simulink library "atomicSubSystem"  (R2023a)
settings: Solver=VariableStepAuto  StartTime=0.0  StopTime=10.0  RelTol=1e-3
libraries: $bdroot x1
settings Model: Creator=Franz  LastModifiedBy=Franz

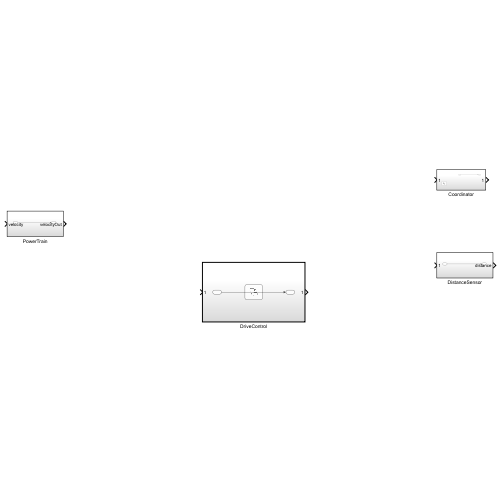
[thumbnail: Simulink's stored preview of the top-level diagram]
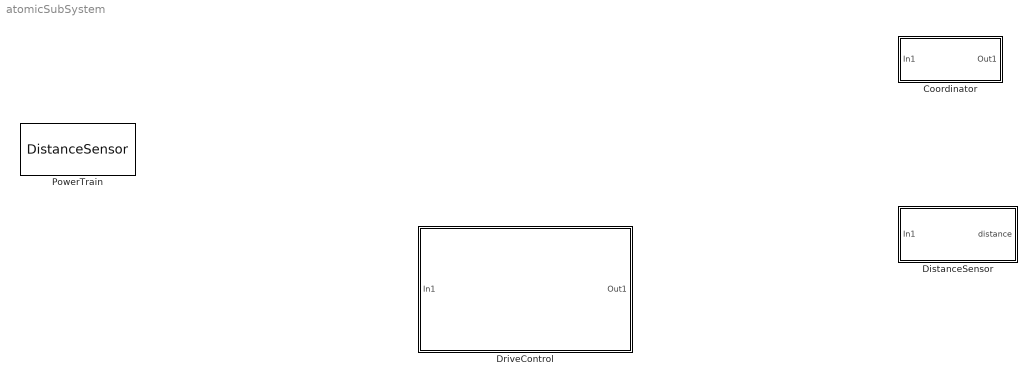
== system atomicSubSystem ==
  Coordinator : Subsystem
  DistanceSensor : Subsystem
  DriveControl : Subsystem  TreatAsAtomicUnit=on
  PowerTrain : $bdroot/DistanceSensor  SystemSampleTime=-1  VariantActivationTime=update diagram  Latency=0  AutoFrameSizeCalculation=off

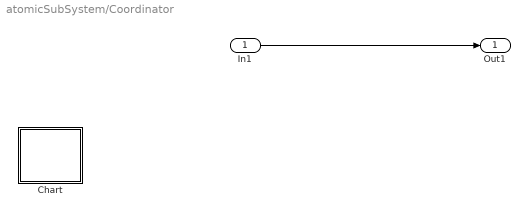
== system atomicSubSystem/Coordinator ==
  In1 : Inport
  Chart : Stateflow chart  TreatAsAtomicUnit=on
  Out1 : Outport
  wires:
  In1/1 -> Out1/1

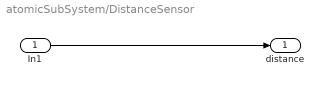
== system atomicSubSystem/DistanceSensor ==
  In1 : Inport
  distance : Outport
  wires:
  In1/1 -> distance/1

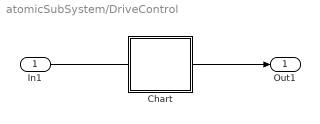
== system atomicSubSystem/DriveControl ==
  In1 : Inport
  Chart : Stateflow chart  TreatAsAtomicUnit=on
  Out1 : Outport
  wires:
  In1/1 -> Out1/1

== stateflow chart atomicSubSystem/DriveControl/Chart ==

== stateflow chart atomicSubSystem/Coordinator/Chart ==
